simulink model "ComunicacionUDP"  (R2020a)
settings: Solver=VariableStepAuto  StartTime=0.0  StopTime=inf  RelTol=1e-3
undefined symbols (not defined in the file): Standard_Devices, UDP_Protocol
libraries: sldrtlib x1
settings Model: Creator=alrer  LastModifiedBy=alrer

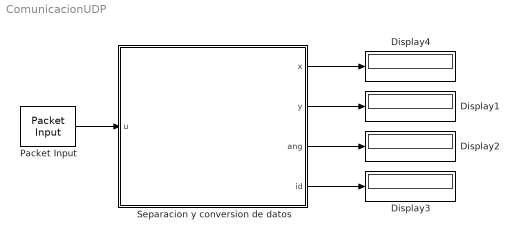
== system ComunicacionUDP ==
  Display{1..4} (4 alike) : Display
  Packet Input : sldrtlib/Packet Input  SampleTime=0.001  MaxMissedTicks=inf  ShowMissedTicks=off  YieldWhenWaiting=off  DrvName=Standard_Devices/UDP_Protocol  DrvAddress=58624  DrvOptions=[0 58624 49 50 55 46 48 46 48 46 49 0 0 0 0 0 0 0 0 0 0 0 0 0 0 0 0 0 0 0 0 0 0 0 0 0 0 0 0 0 0 0 0 0 0 0 0 0 0 0 0 0 0 0 0 0 0 0 0 0 0 0 0 0 0 0 0 0 0 0 0 0 0 0 0 0 0 0 0 0 0 0 0 0 0 0 0 0 0 0 0 0 0 0 0 0 0 0 0 0 0 0 0 0 0 0 0 0 0 0 0 0 0 0 0 0 0 0 0 0 0 0 0 0 0 0 0 0 0 0 0 0 0 0 0 0 0 0 0 0 0 0 0 0 0 0 0 0 0 0 0 0 0 0 0 0 0 0 0 0 0 0 0 0 0 0 0 0 0 0 0 0 0 0 0 0 0 0 0 0 0 0 0 0 0 0 0 0 0 0 0 0 0 0 0 0 0 0 0 0 0 0 0 0 0 0 0 0 0 0 0 0 0 0 0 0 0 0 0 0 0 0 0 0 0 0 0 0 0 0 0 0 0 0 0 0 0 0 0 0 0 0 0 0 0 0 0 0 0 0 0 0 0 0 0 0]  PacketSize=34  DataTypes='34*int8'  ShowReady=off  ShowError=off  PacketID=1  ByteOrder=1  ShowTimestamp=off
      settings: AttributesFormatString=UDP Protocol [58624]
  Separacion y conversion de datos : MATLAB Function  TreatAsAtomicUnit=on
  wires:
  Packet Input/1 -> Separacion y conversion de datos/1(u)
  Separacion y conversion de datos/1(x) -> Display4/1
  Separacion y conversion de datos/2(y) -> Display1/1
  Separacion y conversion de datos/3(ang) -> Display2/1
  Separacion y conversion de datos/4(id) -> Display3/1

== matlab function ComunicacionUDP/Separacion y conversion de datos ==
  data: u input; x output; y output; ang output; id output
function [x, y, ang, id] = fcn(u)
    aux=0;
    e=zeros(17);

    for i=1:1:17
        if u(i)==77 % Identificador de inicio de cadena "M"
            aux=i;
        end
    end
    
    r=17;
    for j=1:1:r
        e(j)=u(aux+j);
    end

    id = e(16)-48;
    x=(e(2)-48)*1000+(e(3)-48)*100+(e(4)-48)*10+(e(5)-48);
    y=(e(7)-48)*1000+(e(8)-48)*100+(e(9)-48)*10+(e(10)-48);
    ang=(e(13)-48)*100 + (e(14)-48)*10 + (e(15)-48);

    if(e(1)==45)
           x = -x;
    end

    if(e(6)==45)
           y = -y;
    end
end
